simulink model "cw1_sim"  (Simulink 8.3)
settings: Solver=ode45  StartTime=tp  StopTime=tk  MaxStep=dtmax  MinStep=dtmin  RelTol=1e-3
values from neighbouring files (symbols this model uses):
  omega = 2*pi*f    (= 314.159265359)    [Scw1_Simulink.m]
  Um = UN*2^0.5    (= 325.269119346)    [Scw1_Simulink.m]
libraries: simulink x1
settings Model: Creator=user  LastModifiedBy=user
settings SolverCC: InitialStep=dtpocz
settings DataIOCC: SignalLoggingSaveFormat=Dataset
settings DebuggingCC: UnderspecifiedInitializationDetection=Simplified  StateNameClashWarn=none
settings GRTTargetCC: CombineOutputUpdateFcns=on  GRTInterface=off

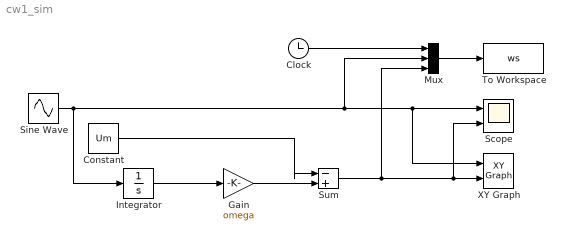
== system cw1_sim ==
  Clock : Clock
  Constant : Constant  Value=Um
  Gain : Gain  Gain=omega
  Integrator : Integrator
  Mux : Mux  Inputs=3
  Scope : Scope  NumInputPorts=2
      settings: YMin=-5~-5  YMax=5~5
  Sine Wave : Sin  Amplitude=Um  Frequency=omega  Phase=fi  SampleTime=0
  Sum : Sum  Inputs=|-+
  To Workspace : ToWorkspace  VariableName=ws  SampleTime=-1
  XY Graph : simulink/Sinks/XY Graph  xmin=-Um  xmax=Um  ymin=-Um  ymax=Um  st=-1
  wires:
  Sine Wave/1 -> Integrator/1, Mux/2, XY Graph/1, Scope/1
  Integrator/1 -> Gain/1
  Gain/1 -> Sum/2
  Constant/1 -> Sum/1
  Sum/1 -> XY Graph/2, Scope/2, Mux/3
  Clock/1 -> Mux/1
  Mux/1 -> To Workspace/1
